simulink model "first"  (R2023a)
settings: Solver=VariableStepAuto  StartTime=0.0  StopTime=180  RelTol=1e-3
settings Model: Creator=eriknymobohne  LastModifiedBy=eriknymobohne

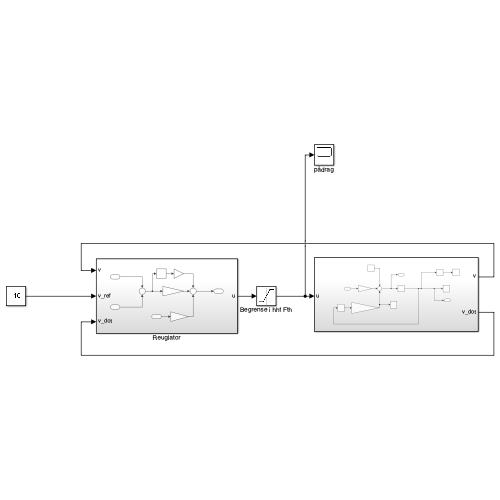
[thumbnail: Simulink's stored preview of the top-level diagram]
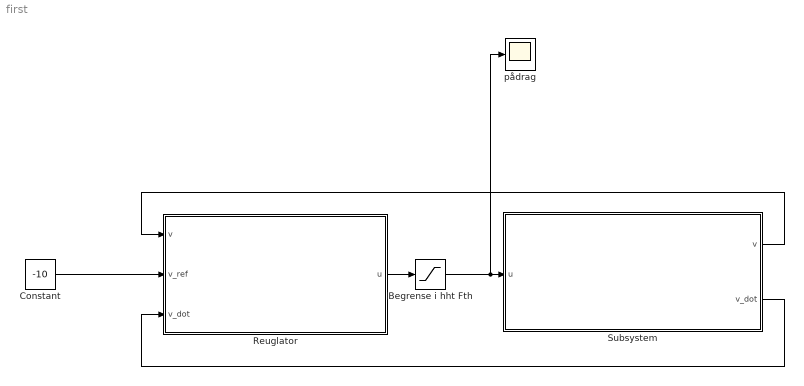
== system first ==
  Begrense i hht Fth : Saturate  UpperLimit=845000*9  LowerLimit=0
  Constant : Constant  Value=-10
  Reuglator : Subsystem
  Subsystem : Subsystem
  pådrag : Scope
  wires:
  Constant/1 -> Reuglator/2(v_ref)
  Subsystem/1(v) -> Reuglator/1(v)
  Subsystem/2(v_dot) -> Reuglator/3(v_dot)
  Reuglator/1(u) -> Begrense i hht Fth/1
  Begrense i hht Fth/1 -> pådrag/1, Subsystem/1(u)

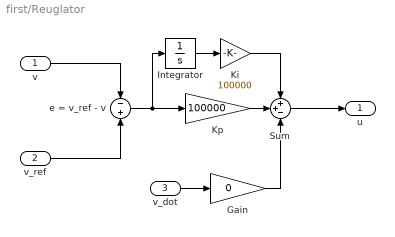
== system first/Reuglator ==
  v : Inport
  v_ref : Inport  Port=2
  v_dot : Inport  Port=3
  Gain : Gain  Gain=0
  Integrator : Integrator
  Ki : Gain  Gain=100000
  Kp : Gain  Gain=100000
  Sum : Sum  Inputs=++-
  e = v_ref - v : Sum  Inputs=-|+
  u : Outport
  wires:
  v_ref/1 -> e = v_ref - v/2
  v/1 -> e = v_ref - v/1
  e = v_ref - v/1 -> Kp/1, Integrator/1
  Sum/1 -> u/1
  Kp/1 -> Sum/2
  Integrator/1 -> Ki/1
  Ki/1 -> Sum/1
  v_dot/1 -> Gain/1
  Gain/1 -> Sum/3

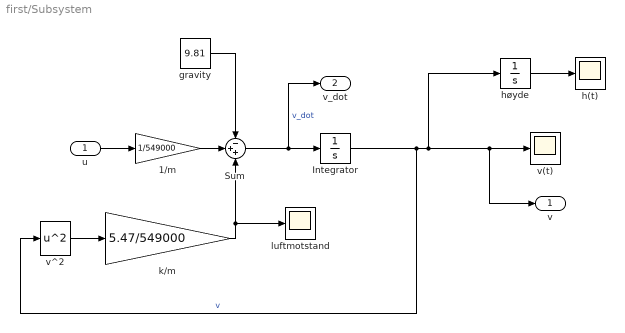
== system first/Subsystem ==
  u : Inport
  1/m : Gain  Gain=1/549000
  Integrator : Integrator  InitialCondition=-1000
  Sum : Sum  Inputs=-++
  gravity : Constant  Value=9.81
  h(t) : Scope
  høyde : Integrator  InitialCondition=10000
  k/m : Gain  Gain=5.47/549000
  luftmotstand : Scope
  v(t) : Scope
  v^2 : Math  Operator=square
  v : Outport
  v_dot : Outport  Port=2
  wires:
  Integrator/1 -> v^2/1, høyde/1, v/1, v(t)/1  "v"
  gravity/1 -> Sum/1
  Sum/1 -> v_dot/1, Integrator/1  "v_dot"
  v^2/1 -> k/m/1
  k/m/1 -> luftmotstand/1, Sum/3
  høyde/1 -> h(t)/1
  1/m/1 -> Sum/2
  u/1 -> 1/m/1
